simulink model "sampleModel153_pp_1136_1"  (R2021a)
settings: Solver=VariableStepAuto  StartTime=0.0  StopTime=10.0  RelTol=1e-3
undefined symbols (not defined in the file or in its folder): DiscIntNeverNeededParam, magnitude, Newton, Raphson
libraries: simulink x48, pid_lib x19
(part 1 of 3)
settings Model: Creator=CMelt  LastModifiedBy=user

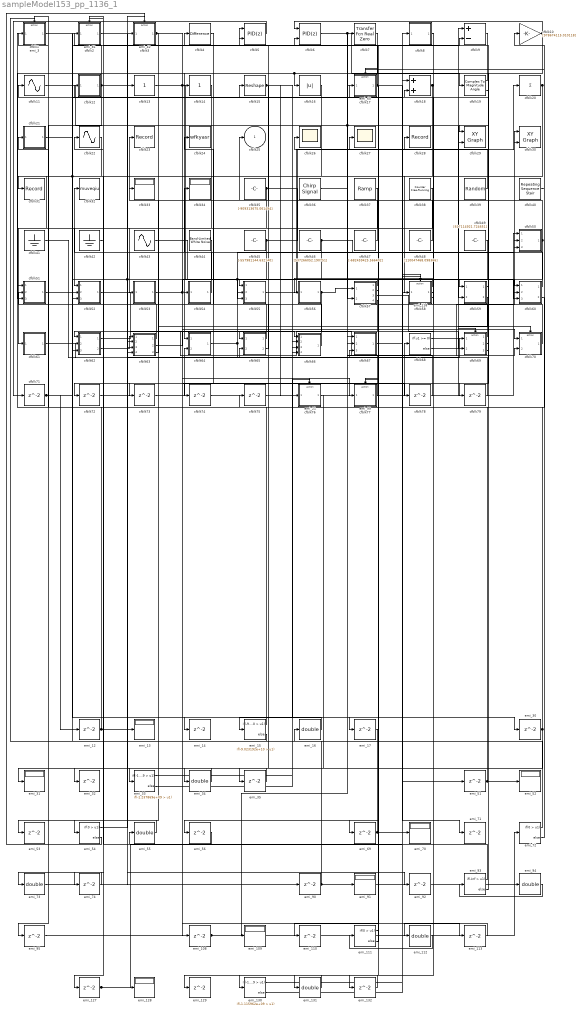
== system sampleModel153_pp_1136_1 ==
  cfblk1 : Subsystem  TreatAsAtomicUnit=on
  cfblk10 : Gain  Gain=[978674115.010118]
  cfblk11 : Sin  TimeSource=Use external signal  SampleTime=0
  cfblk12 : Subsystem  TreatAsAtomicUnit=on
  cfblk13 : simulink/Math Operations/Slider Gain  gain=1  low=0  high=2
  cfblk14 : simulink/Math Operations/Slider Gain  gain=1  low=0  high=2
  cfblk15 : Reshape
  cfblk16 : Abs
  cfblk17 : Subsystem  TreatAsAtomicUnit=on
  cfblk18 : Sum
  cfblk19 : ComplexToMagnitudeAngle
  cfblk2 : Subsystem  TreatAsAtomicUnit=on
  cfblk20 : Sum  Inputs=+
  cfblk21 : Subsystem  TreatAsAtomicUnit=on
  cfblk22 : Sin  TimeSource=Use external signal  SampleTime=0
  cfblk23 : Record  FileSettingsInternal="{\"entries\":[{\"content\":{\"excelSettings\":{\"content\":{},\"type\":\"Streamout.ExcelSettings\"}},\"type\":\"Streamout.FileSettingStorage\",\"uuid\":\"90d3bf4d-074c-419f-bc98-93890882def7\"}],\"packageUris\":[\"http://schema.mathworks.com/mf0/streamout_blocks/R2020a\"],\"version\":\"1.0\"}"  SignalsInternal="{\"entries\":[{\"content\":{\"signals\":[{\"content\":{\"blockPath\":[\"sampleModel153_pp_1136_1/cfblk23\"],\"channel\":[],\"dimensions\":[1],\"domain\":\"samplemodel153_pp_1136_1/cfblk23\",\"lineColor\":\"#64d413\",\"plots\":[1],\"port\":1,\"sid\":[\"\"],\"signalID\":1445323,\"signalName\":\"cfblk47\"},\"type\":\"RecordBlkView.Signal\",\"uuid\":\"54714383-f197-4a3d-9991-f85be281b323\"}]},\"type\":\"RecordBlkView.InputSignals\",\"uuid\":\"544324a9-3e37-4335-a052-9c5c4b19bc85\"}],\"packageUris\":[\"http://schema.mathworks.com/mf0/streamout_blocks/R2020a\"],\"version\":\"1.0\"}"  VisualizationBindings="{\"sparklinesplugin\":{\"info\":[{\"bindingParametersList\":[],\"subplotID\":1}]}}"
  cfblk24 : ToWorkspace  VariableName=wfkyasr  SaveFormat=Timeseries  SampleTime=-1
  cfblk26 : Scope
  cfblk27 : Scope
  cfblk28 : Record  FileSettingsInternal="{\"entries\":[{\"content\":{\"excelSettings\":{\"content\":{},\"type\":\"Streamout.ExcelSettings\"}},\"type\":\"Streamout.FileSettingStorage\",\"uuid\":\"e040c9fa-48bd-4228-9996-6934888816c0\"}],\"packageUris\":[\"http://schema.mathworks.com/mf0/streamout_blocks/R2020a\"],\"version\":\"1.0\"}"  SignalsInternal="{\"entries\":[{\"content\":{\"signals\":[{\"content\":{\"blockPath\":[\"sampleModel153_pp_1136_1/cfblk28\"],\"channel\":[],\"dimensions\":[1],\"domain\":\"samplemodel153_pp_1136_1/cfblk28\",\"lineColor\":\"#a2142f\",\"plots\":[1],\"port\":1,\"sid\":[\"\"],\"signalID\":1445307,\"signalName\":\"cfblk70\"},\"type\":\"RecordBlkView.Signal\",\"uuid\":\"60194e6e-711a-4c83-acfc-41706555a870\"}]},\"type\":\"RecordBlkView.InputSignals\",\"uuid\":\"f9cd218e-cda2-4dab-b38f-344dbdd6f2d9\"}],\"packageUris\":[\"http://schema.mathworks.com/mf0/streamout_blocks/R2020a\"],\"version\":\"1.0\"}"  VisualizationBindings="{\"sparklinesplugin\":{\"info\":[{\"bindingParametersList\":[],\"subplotID\":1}]}}"
  cfblk29 : simulink/Sinks/XY Graph  xmin=-1  xmax=1  ymin=-1  ymax=1  st=-1
  cfblk3 : Subsystem  TreatAsAtomicUnit=on
  cfblk30 : simulink/Sinks/XY Graph  xmin=-1  xmax=1  ymin=-1  ymax=1  st=-1
  cfblk31 : Record  FileSettingsInternal="{\"entries\":[{\"content\":{\"excelSettings\":{\"content\":{},\"type\":\"Streamout.ExcelSettings\"}},\"type\":\"Streamout.FileSettingStorage\",\"uuid\":\"d257a69d-5f58-45b3-980e-d66c6de6435d\"}],\"packageUris\":[\"http://schema.mathworks.com/mf0/streamout_blocks/R2020a\"],\"version\":\"1.0\"}"  SignalsInternal="{\"entries\":[{\"content\":{\"signals\":[{\"content\":{\"blockPath\":[\"sampleModel153_pp_1136_1/cfblk31\"],\"channel\":[],\"dimensions\":[1],\"domain\":\"samplemodel153_pp_1136_1/cfblk31\",\"lineColor\":\"#139fff\",\"plots\":[1],\"port\":1,\"sid\":[\"\"],\"signalID\":1445311,\"signalName\":\"cfblk22\"},\"type\":\"RecordBlkView.Signal\",\"uuid\":\"a9ae145c-d94a-4c8d-ae8c-213f4e7c6313\"}]},\"type\":\"RecordBlkView.InputSignals\",\"uuid\":\"9bb384fc-6cf1-475e-b446-87fd7b0246af\"}],\"packageUris\":[\"http://schema.mathworks.com/mf0/streamout_blocks/R2020a\"],\"version\":\"1.0\"}"  VisualizationBindings="{\"sparklinesplugin\":{\"info\":[{\"bindingParametersList\":[],\"subplotID\":1}]}}"
  cfblk32 : ToWorkspace  VariableName=muveqiu  SaveFormat=Timeseries  SampleTime=-1
  cfblk33 : Display
  cfblk34 : Display
  cfblk35 : Constant  Value=[-909313675.061494]  SampleTime=1
  cfblk36 : simulink/Sources/Chirp Signal  f1=[222988645.109362]  T=[-499288554.133847]  f2=[-768297567.598976]
  cfblk37 : simulink/Sources/Ramp  slope=[-4243.323419]  start=[2.640066]  InitialOutput=[-454218.144588]
  cfblk38 : simulink/Sources/Counter Free-Running  NumBits=[41.000000]  tsamp=-1
  cfblk39 : RandomNumber  Mean=[50925.059613]  Variance=[74743.961687]  Seed=[936037609.000000]  SampleTime=0.1
  cfblk4 : simulink/Discrete/Difference  ICPrevInput=0.0  OutMin=[]  OutMax=[]  OutDataTypeStr=Inherit: Inherit via back propagation  OutDataType=fixdt(1, 16)  OutScaling=2^-10  DoSatur=off
  cfblk40 : simulink/Sources/Repeating Sequence Stair  OutValues=[20471336.287258, 516776994.362484]  tsamp=-1  OutMin=[]  OutMax=[]  OutDataTypeStr=double  OutputDataTypeScalingMode=double  OutDataType=fixdt(0,8)  ConRadixGroup=Best Precision: Vector-wise  OutScaling=2^-12
  cfblk41 : Ground
  cfblk42 : Ground
  cfblk43 : Sin  Amplitude=[411017869.631125]  Bias=[-642889720.785330]  SampleTime=0
  cfblk44 : simulink/Sources/Band-Limited White Noise  Cov=[8221267165.313615]  Ts=0.1  seed=[5325572605.000000]
  cfblk45 : Constant  Value=[-557981144.632140]  SampleTime=1
  cfblk46 : Constant  Value=[537266052.190751]  SampleTime=1
  cfblk47 : Constant  Value=[-682459425.566402]  SampleTime=1
  cfblk48 : Constant  Value=[110047468.098366]  SampleTime=1
  cfblk49 : Constant  Value=[617114921.724651]  SampleTime=1
  cfblk5 : pid_lib/PID Controller (2DOF)  Controller=PID  Form=Parallel  TimeDomain=Discrete-time  UseExternalTs=off  SampleTime=1  IntegratorMethod=Forward Euler  FilterMethod=Forward Euler  ControllerParametersSource=internal  P=1  I=1  D=0  UseFilter=on  N=100  b=1  c=1  TunerSelectOption=Transfer Function Based (PID Tuner App)  InitialConditionSource=internal  InitialConditionForIntegrator=0  InitialConditionForFilter=0  DifferentiatorICPrevScaledInput=0  ExternalReset=none  TrackingMode=off  Kt=1  LimitOutput=off  SatLimitsSource=internal  UpperSaturationLimit=inf  LowerSaturationLimit=-inf  LinearizeAsGain=off  AntiWindupMode=none  Kb=1  POutMin=[]  POutMax=[]  IOutMin=[]  IOutMax=[]  DOutMin=[]  DOutMax=[]  NOutMin=[]  NOutMax=[]  bOutMin=[]  bOutMax=[]  cOutMin=[]  cOutMax=[]  SumOutMin=[]  SumOutMax=[]  SaturationOutMin=[]  SaturationOutMax=[]  PParamMin=[]  PParamMax=[]  IParamMin=[]  IParamMax=[]  DParamMin=[]  DParamMax=[]  NParamMin=[]  NParamMax=[]  bParamMin=[]  bParamMax=[]  cParamMin=[]  cParamMax=[]  KbParamMin=[]  KbParamMax=[]  KtParamMin=[]  KtParamMax=[]  KbOutMin=[]  KbOutMax=[]  KtOutMin=[]  KtOutMax=[]  IntegratorOutMin=[]  IntegratorOutMax=[]  FilterOutMin=[]  FilterOutMax=[]  SumI1OutMin=[]  SumI1OutMax=[]  SumI2OutMin=[]  SumI2OutMax=[]  SumI3OutMin=[]  SumI3OutMax=[]  SumI4OutMin=[]  SumI4OutMax=[]  SumDOutMin=[]  SumDOutMax=[]  Sum1OutMin=[]  Sum1OutMax=[]  Sum2OutMin=[]  Sum2OutMax=[]  Sum3OutMin=[]  Sum3OutMax=[]  DifferentiatorOutMin=[]  DifferentiatorOutMax=[]  FilterDiffOutCoefMin=[]  FilterDiffOutCoefMax=[]  ReciprocalOutMin=[]  ReciprocalOutMax=[]  SumDenOutMin=[]  SumDenOutMax=[]  SumNumOutMin=[]  SumNumOutMax=[]  DivideOutMin=[]  DivideOutMax=[]  UdiffTsProdOutMin=[]  UdiffTsProdOutMax=[]  NTsProdOutMin=[]  NTsProdOutMax=[]  UintegralTsProdOutMin=[]  UintegralTsProdOutMax=[]  UngainTsProdOutMin=[]  UngainTsProdOutMax=[]  IntegratorContinuousStateAttributes=''  IntegratorStateMustResolveToSignalObject=off  IntegratorRTWStateStorageClass=Auto  FilterContinuousStateAttributes=''  FilterStateMustResolveToSignalObject=off  FilterRTWStateStorageClass=Auto  ParallelPVariant=InternalParameters  IdealPVariant=Disabled  IVariant=InternalParameters  DVariant=InternalParameters  bVariant=InternalParameters  cVariant=InternalParameters  IntegratorVariant=Discrete  SatVariant=Disabled  AWVariant=Passthrough  PCopyVariant=Disabled  TRVariant=Disabled  FdbkBlocksVariant=Forward  IdealPFdbkVariant=Disabled  SatFdbkVariant=Disabled  DerivativeFilterVariant=ForwardEulerFilter  NVariant=InternalParameters  NCopyVariant=Disabled  FilterICVariant=InternalICsFilter  IntegratorICVariant=InternalICs  ExternalResetVariant=Disabled  TRSumVariant=Passthrough  SumFdbkVariant=Disabled  SumVariant=Sum_PID  TsampFilterVariant=InternalTs  TsampNgainVariant=Passthrough  TsampIntegralVariant=Passthrough  ExternalSaturationOutDataTypeStr=Inherit: Same as second input
      settings: SourceProductBaseCode=SL
  cfblk50 : Subsystem
  cfblk51 : Subsystem
  cfblk52 : Subsystem
  cfblk53 : Subsystem
  cfblk54 : Subsystem
  cfblk55 : Subsystem
  cfblk56 : Subsystem
  cfblk57 : Subsystem
  cfblk58 : Subsystem  TreatAsAtomicUnit=on
  cfblk59 : Subsystem
  cfblk6 : pid_lib/PID Controller (2DOF)  Controller=PID  Form=Parallel  TimeDomain=Discrete-time  UseExternalTs=off  SampleTime=1  IntegratorMethod=Forward Euler  FilterMethod=Forward Euler  ControllerParametersSource=internal  P=1  I=1  D=0  UseFilter=on  N=100  b=1  c=1  TunerSelectOption=Transfer Function Based (PID Tuner App)  InitialConditionSource=internal  InitialConditionForIntegrator=0  InitialConditionForFilter=0  DifferentiatorICPrevScaledInput=0  ExternalReset=none  TrackingMode=off  Kt=1  LimitOutput=off  SatLimitsSource=internal  UpperSaturationLimit=inf  LowerSaturationLimit=-inf  LinearizeAsGain=off  AntiWindupMode=none  Kb=1  POutMin=[]  POutMax=[]  IOutMin=[]  IOutMax=[]  DOutMin=[]  DOutMax=[]  NOutMin=[]  NOutMax=[]  bOutMin=[]  bOutMax=[]  cOutMin=[]  cOutMax=[]  SumOutMin=[]  SumOutMax=[]  SaturationOutMin=[]  SaturationOutMax=[]  PParamMin=[]  PParamMax=[]  IParamMin=[]  IParamMax=[]  DParamMin=[]  DParamMax=[]  NParamMin=[]  NParamMax=[]  bParamMin=[]  bParamMax=[]  cParamMin=[]  cParamMax=[]  KbParamMin=[]  KbParamMax=[]  KtParamMin=[]  KtParamMax=[]  KbOutMin=[]  KbOutMax=[]  KtOutMin=[]  KtOutMax=[]  IntegratorOutMin=[]  IntegratorOutMax=[]  FilterOutMin=[]  FilterOutMax=[]  SumI1OutMin=[]  SumI1OutMax=[]  SumI2OutMin=[]  SumI2OutMax=[]  SumI3OutMin=[]  SumI3OutMax=[]  SumI4OutMin=[]  SumI4OutMax=[]  SumDOutMin=[]  SumDOutMax=[]  Sum1OutMin=[]  Sum1OutMax=[]  Sum2OutMin=[]  Sum2OutMax=[]  Sum3OutMin=[]  Sum3OutMax=[]  DifferentiatorOutMin=[]  DifferentiatorOutMax=[]  FilterDiffOutCoefMin=[]  FilterDiffOutCoefMax=[]  ReciprocalOutMin=[]  ReciprocalOutMax=[]  SumDenOutMin=[]  SumDenOutMax=[]  SumNumOutMin=[]  SumNumOutMax=[]  DivideOutMin=[]  DivideOutMax=[]  UdiffTsProdOutMin=[]  UdiffTsProdOutMax=[]  NTsProdOutMin=[]  NTsProdOutMax=[]  UintegralTsProdOutMin=[]  UintegralTsProdOutMax=[]  UngainTsProdOutMin=[]  UngainTsProdOutMax=[]  IntegratorContinuousStateAttributes=''  IntegratorStateMustResolveToSignalObject=off  IntegratorRTWStateStorageClass=Auto  FilterContinuousStateAttributes=''  FilterStateMustResolveToSignalObject=off  FilterRTWStateStorageClass=Auto  ParallelPVariant=InternalParameters  IdealPVariant=Disabled  IVariant=InternalParameters  DVariant=InternalParameters  bVariant=InternalParameters  cVariant=InternalParameters  IntegratorVariant=Discrete  SatVariant=Disabled  AWVariant=Passthrough  PCopyVariant=Disabled  TRVariant=Disabled  FdbkBlocksVariant=Forward  IdealPFdbkVariant=Disabled  SatFdbkVariant=Disabled  DerivativeFilterVariant=ForwardEulerFilter  NVariant=InternalParameters  NCopyVariant=Disabled  FilterICVariant=InternalICsFilter  IntegratorICVariant=InternalICs  ExternalResetVariant=Disabled  TRSumVariant=Passthrough  SumFdbkVariant=Disabled  SumVariant=Sum_PID  TsampFilterVariant=InternalTs  TsampNgainVariant=Passthrough  TsampIntegralVariant=Passthrough  ExternalSaturationOutDataTypeStr=Inherit: Same as second input
      settings: SourceProductBaseCode=SL
  cfblk60 : Subsystem
  cfblk61 : Subsystem
  cfblk62 : Subsystem
  cfblk63 : Subsystem
  cfblk64 : Subsystem
  cfblk65 : Subsystem
  cfblk66 : Subsystem
  cfblk67 : Subsystem
  cfblk68 : If  IfExpression=u1 >= 0  SampleTime=1
  cfblk69 : Subsystem  TreatAsAtomicUnit=on
  cfblk7 : simulink/Discrete/Transfer Fcn Real Zero  ZeroZ=0.75  ICPrevInput=0.0  DoSatur=off
      settings: SourceProductBaseCode=SL
  cfblk70 : Subsystem  TreatAsAtomicUnit=on
  cfblk{71..75,78..79} (7 alike) : Delay  SampleTime=1
  cfblk76 : Subsystem  TreatAsAtomicUnit=on
  cfblk77 : Subsystem  TreatAsAtomicUnit=on
  cfblk8 : ModelReference  ModelNameDialog=sampleModel_ref_684  SimulationMode=Normal  ModelReferenceVersion=1.1
  cfblk9 : Sum  Inputs=+-
  emi_{12,14,30,32,90,92,108,110} (8 alike) : Delay
  emi_{13,31,52,70,91,109,128} (7 alike) : Display
  emi_111 : If  IfExpression=0 > u1  SampleTime=1
  emi_{16,34,55,73,94,112,131} (7 alike) : DataTypeConversion  OutDataTypeStr=double
  emi_113 : Delay  InitialCondition=0
  emi_118 : Subsystem  TreatAsAtomicUnit=on
  emi_{51,53,69,71,127,129} (6 alike) : Delay  SampleTime=1
  emi_130 : If  IfExpression=-1.115962e+09 > u1
  emi_132 : Delay  InitialCondition=-557981144.6321
  emi_15 : If  IfExpression=-9.023192e+10 > u1  SampleTime=1
  emi_17 : Delay  InitialCondition=-45115958295.9639
  emi_21 : Subsystem  TreatAsAtomicUnit=on
  emi_3 : Subsystem  TreatAsAtomicUnit=on
  emi_33 : If  IfExpression=-1.237869e+09 > u1  SampleTime=1
  emi_35 : Delay  InitialCondition=-618934691.025
  emi_42 : Subsystem  TreatAsAtomicUnit=on
  emi_54 : If  IfExpression=0 > u1  SampleTime=1
  emi_56 : Delay  InitialCondition=0
  emi_60 : Subsystem  TreatAsAtomicUnit=on
  emi_72 : If  IfExpression=0 > u1
  emi_74 : Delay  InitialCondition=0
  emi_81 : Subsystem  TreatAsAtomicUnit=on
  emi_93 : If  IfExpression=-Inf > u1
  emi_95 : Delay  InitialCondition=-Inf
  emi_99 : Subsystem  TreatAsAtomicUnit=on
  cfblk25 : Outport
  wires:
  cfblk9/1 -> cfblk64/1(cfblk1)
  cfblk47/1 -> cfblk23/1
  cfblk38/1 -> cfblk52/1(cfblk1)
  cfblk57/1(cfblk2) -> cfblk52/2(cfblk8)
  cfblk41/1 -> cfblk69/1(cfblk1)
  cfblk39/1 -> cfblk27/1
  cfblk49/1 -> cfblk54/1(cfblk1)
  cfblk62/1(cfblk2) -> cfblk30/1
  cfblk63/2(cfblk15) -> cfblk66/1(cfblk1)
  cfblk35/1 -> cfblk61/1(cfblk1), cfblk60/2(cfblk10)
  cfblk57/2(cfblk12) -> cfblk11/1
  cfblk22/1 -> cfblk31/1
  cfblk6/1 -> cfblk29/2, cfblk60/3(cfblk11), cfblk19/1
  cfblk48/1 -> cfblk25/1
  cfblk70/1(cfblk2) -> cfblk28/1
  cfblk62/2(cfblk11) -> cfblk63/1(cfblk1)
  cfblk46/1 -> cfblk52/3(cfblk9), cfblk55/3(cfblk12), cfblk50/3(cfblk14)
  cfblk52/1(cfblk2) -> cfblk65/1(cfblk1)
  cfblk13/1 -> cfblk55/1(cfblk1), cfblk70/1(cfblk1)
  cfblk36/1 -> cfblk7/1
  cfblk63/3(cfblk16) -> cfblk33/1
  cfblk54/1(cfblk2) -> cfblk32/1
  cfblk61/1(cfblk2) -> cfblk65/2(cfblk6)
  cfblk19/1 -> cfblk14/1
  cfblk10/1 -> cfblk6/1, cfblk29/1
  cfblk14/1 -> cfblk53/1(cfblk1)
  cfblk66/1(cfblk2) -> cfblk24/1
  cfblk65/1(cfblk2) -> cfblk22/1
  cfblk16/1 -> cfblk51/1(cfblk1), cfblk62/3(cfblk10)
  cfblk37/1 -> cfblk66/2(cfblk12)
  cfblk60/1(cfblk2) -> cfblk34/1
  cfblk7/1 -> cfblk16/1, cfblk51/3(cfblk7)
  cfblk65/2(cfblk7) -> cfblk51/2(cfblk6)
  cfblk57/3(cfblk13) -> cfblk69/2(cfblk10)
  cfblk69/1(cfblk2) -> cfblk4/1
  cfblk53/1(cfblk2) -> cfblk59/1(cfblk1), cfblk78/1
  cfblk11/1 -> cfblk59/2(cfblk6)
  cfblk56/1(cfblk2) -> cfblk57/1(cfblk1), cfblk63/4(cfblk14)
  cfblk55/1(cfblk2) -> cfblk30/2
  cfblk51/1(cfblk2) -> cfblk5/1
  cfblk44/1 -> cfblk63/3(cfblk13), cfblk62/2(cfblk9)
  cfblk69/2(cfblk11) -> cfblk15/1
  cfblk69/3(cfblk12) -> cfblk26/1
  cfblk15/1 -> cfblk60/1(cfblk1), cfblk76/1(emi_19), emi_30/1, emi_35/1
  cfblk40/1 -> cfblk10/1
  cfblk43/1 -> cfblk66/3(cfblk13)
  cfblk64/1(cfblk2) -> cfblk50/2(cfblk13), cfblk67/3(cfblk7)
  cfblk45/1 -> cfblk55/2(cfblk11), cfblk20/1
  cfblk57/4(cfblk14) -> cfblk66/4(cfblk14)
  cfblk50/1(cfblk2) -> cfblk57/2(cfblk11), cfblk5/2
  cfblk68/1 -> cfblk69/Action
  cfblk68/2 -> cfblk70/Action
  cfblk5/1 -> cfblk71/1
  cfblk59/1(cfblk2) -> cfblk72/1
  cfblk72/1 -> cfblk64/2(cfblk7)
  cfblk59/2(cfblk7) -> cfblk73/1
  cfblk73/1 -> cfblk9/1
  cfblk4/1 -> cfblk74/1
  cfblk74/1 -> cfblk68/1
  cfblk60/2(cfblk12) -> cfblk75/1
  cfblk75/1 -> cfblk50/1(cfblk1)
  cfblk78/1 -> cfblk67/2(cfblk6)
  cfblk19/2 -> cfblk79/1
  cfblk79/1 -> cfblk63/2(cfblk12)
  cfblk71/1 -> cfblk1/1(emi_1), emi_12/1, emi_17/1
  cfblk1/1(emi_2) -> cfblk9/2
  emi_12/1 -> emi_3/1(emi_10), emi_13/1
  emi_3/1(emi_11) -> emi_14/1
  emi_15/2 -> cfblk1/Action
  emi_15/1 -> emi_3/Action
  emi_16/1 -> emi_15/1
  emi_17/1 -> emi_16/1
  cfblk76/1(emi_20) -> cfblk70/2(cfblk9)
  emi_30/1 -> emi_21/1(emi_28), emi_31/1
  emi_21/1(emi_29) -> emi_32/1
  emi_33/2 -> cfblk76/Action
  emi_33/1 -> emi_21/Action
  emi_34/1 -> emi_33/1
  emi_35/1 -> emi_34/1
  cfblk42/1 -> cfblk12/1(emi_37)
  cfblk3/1(emi_41) -> cfblk6/2, cfblk77/1(emi_97), emi_108/1, emi_113/1
  emi_51/1 -> emi_42/1(emi_49), emi_52/1
  emi_42/1(emi_50) -> emi_53/1
  emi_54/2 -> cfblk3/Action
  emi_54/1 -> emi_42/Action
  emi_55/1 -> emi_54/1
  emi_56/1 -> emi_55/1
  cfblk18/1 -> cfblk17/1(emi_58), emi_69/1, emi_74/1
  cfblk17/1(emi_59) -> emi_56/1, emi_51/1, cfblk3/1(emi_40)
  emi_69/1 -> emi_60/1(emi_67), emi_70/1
  emi_60/1(emi_68) -> emi_71/1
  emi_72/2 -> cfblk17/Action
  emi_72/1 -> emi_60/Action
  emi_73/1 -> emi_72/1
  emi_74/1 -> emi_73/1
  cfblk63/1(cfblk2) -> cfblk21/1(emi_76)
  cfblk21/1(emi_77) -> cfblk18/1
  cfblk12/1(emi_38) -> cfblk2/1(emi_79), emi_90/1, emi_95/1
  cfblk2/1(emi_80) -> cfblk13/1
  emi_90/1 -> emi_81/1(emi_88), emi_91/1
  emi_81/1(emi_89) -> emi_92/1
  emi_93/2 -> cfblk2/Action
  emi_93/1 -> emi_81/Action
  emi_94/1 -> emi_93/1
  emi_95/1 -> emi_94/1
  cfblk77/1(emi_98) -> cfblk67/1(cfblk1)
  emi_108/1 -> emi_99/1(emi_106), emi_109/1
  emi_99/1(emi_107) -> emi_110/1
  emi_111/2 -> cfblk77/Action
  emi_111/1 -> emi_99/Action
  emi_112/1 -> emi_111/1
  emi_113/1 -> emi_112/1
  cfblk20/1 -> cfblk58/1(emi_115), emi_127/1, emi_132/1
  cfblk58/1(emi_116) -> cfblk56/1(cfblk1)
  cfblk58/2(emi_117) -> cfblk18/2
  emi_127/1 -> emi_118/1(emi_125), emi_128/1
  emi_118/1(emi_126) -> emi_129/1
  emi_130/2 -> cfblk58/Action
  emi_130/1 -> emi_118/Action
  emi_131/1 -> emi_130/1
  emi_132/1 -> emi_131/1
  cfblk67/1(cfblk2) -> cfblk8/1
  cfblk8/1 -> cfblk62/1(cfblk1)

== system sampleModel153_pp_1136_1/cfblk1 ==
  emi_1 : Inport
  Action Port : ActionPort  ActionPortLabel=else
  cfblk1 : DiscreteFir  SampleTime=1
  emi_2 : Outport
  wires:
  emi_1/1 -> cfblk1/1
  cfblk1/1 -> emi_2/1

== system sampleModel153_pp_1136_1/cfblk12 ==
  emi_37 : Inport  Partition=on  PartitionDimension=1  PartitionWidth=1  PartitionOffset=0
  For Each : ForEach  DisableCoverage=on
  cfblk12 : Math  Operator=log10  SaturateOnIntegerOverflow=on
  emi_38 : Outport  ConcatenationDimension=1
  wires:
  emi_37/1 -> cfblk12/1
  cfblk12/1 -> emi_38/1

== system sampleModel153_pp_1136_1/cfblk17 ==
  emi_58 : Inport
  Action Port : ActionPort  ActionPortLabel=else
  cfblk17 : Signum
  emi_59 : Outport
  wires:
  emi_58/1 -> cfblk17/1
  cfblk17/1 -> emi_59/1

== system sampleModel153_pp_1136_1/cfblk2 ==
  emi_79 : Inport
  Action Port : ActionPort  ActionPortLabel=else
  cfblk2 : simulink/Discrete/Difference  ICPrevInput=0.0  OutMin=[]  OutMax=[]  OutDataTypeStr=Inherit: Inherit via back propagation  OutDataType=fixdt(1, 16)  OutScaling=2^-10  DoSatur=off
  emi_80 : Outport
  wires:
  emi_79/1 -> cfblk2/1
  cfblk2/1 -> emi_80/1

== system sampleModel153_pp_1136_1/cfblk21 ==
  emi_76 : Inport  Partition=on  PartitionDimension=1  PartitionWidth=1  PartitionOffset=0
  For Each : ForEach  DisableCoverage=on
  cfblk21 : Rounding
  emi_77 : Outport  ConcatenationDimension=1
  wires:
  emi_76/1 -> cfblk21/1
  cfblk21/1 -> emi_77/1

== system sampleModel153_pp_1136_1/cfblk3 ==
  emi_40 : Inport
  Action Port : ActionPort  ActionPortLabel=else
  cfblk3 : DiscreteFilter  SampleTime=1
  emi_41 : Outport
  wires:
  emi_40/1 -> cfblk3/1
  cfblk3/1 -> emi_41/1

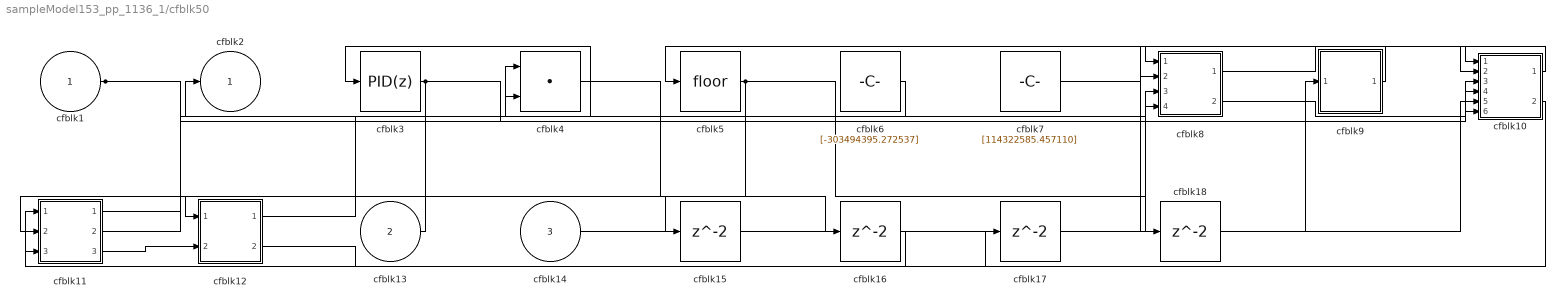
== system sampleModel153_pp_1136_1/cfblk50 ==
  cfblk1 : Inport
  cfblk13 : Inport  Port=2
  cfblk14 : Inport  Port=3
  cfblk10 : Subsystem
  cfblk11 : Subsystem
  cfblk12 : Subsystem
  cfblk{15..18} (4 alike) : Delay  SampleTime=1
  cfblk3 : pid_lib/PID Controller  Controller=PID  Form=Parallel  TimeDomain=Discrete-time  UseExternalTs=off  SampleTime=1  IntegratorMethod=Forward Euler  FilterMethod=Forward Euler  ControllerParametersSource=internal  P=1  I=1  D=0  UseFilter=on  N=100  TunerSelectOption=Transfer Function Based (PID Tuner App)  InitialConditionSource=internal  InitialConditionForIntegrator=0  InitialConditionForFilter=0  DifferentiatorICPrevScaledInput=0  ExternalReset=none  TrackingMode=off  Kt=1  LimitOutput=off  SatLimitsSource=internal  UpperSaturationLimit=inf  LowerSaturationLimit=-inf  LinearizeAsGain=off  AntiWindupMode=none  Kb=1  POutMin=[]  POutMax=[]  IOutMin=[]  IOutMax=[]  DOutMin=[]  DOutMax=[]  NOutMin=[]  NOutMax=[]  SumOutMin=[]  SumOutMax=[]  SaturationOutMin=[]  SaturationOutMax=[]  PParamMin=[]  PParamMax=[]  IParamMin=[]  IParamMax=[]  DParamMin=[]  DParamMax=[]  NParamMin=[]  NParamMax=[]  KbParamMin=[]  KbParamMax=[]  KtParamMin=[]  KtParamMax=[]  KbOutMin=[]  KbOutMax=[]  KtOutMin=[]  KtOutMax=[]  IntegratorOutMin=[]  IntegratorOutMax=[]  FilterOutMin=[]  FilterOutMax=[]  SumI1OutMin=[]  SumI1OutMax=[]  SumI2OutMin=[]  SumI2OutMax=[]  SumI3OutMin=[]  SumI3OutMax=[]  SumI4OutMin=[]  SumI4OutMax=[]  SumDOutMin=[]  SumDOutMax=[]  DifferentiatorOutMin=[]  DifferentiatorOutMax=[]  FilterDiffOutCoefMin=[]  FilterDiffOutCoefMax=[]  ReciprocalOutMin=[]  ReciprocalOutMax=[]  SumDenOutMin=[]  SumDenOutMax=[]  SumNumOutMin=[]  SumNumOutMax=[]  DivideOutMin=[]  DivideOutMax=[]  UdiffTsProdOutMin=[]  UdiffTsProdOutMax=[]  NTsProdOutMin=[]  NTsProdOutMax=[]  UintegralTsProdOutMin=[]  UintegralTsProdOutMax=[]  UngainTsProdOutMin=[]  UngainTsProdOutMax=[]  IntegratorContinuousStateAttributes=''  IntegratorStateMustResolveToSignalObject=off  IntegratorRTWStateStorageClass=Auto  FilterContinuousStateAttributes=''  FilterStateMustResolveToSignalObject=off  FilterRTWStateStorageClass=Auto  ParallelPVariant=InternalParameters  IdealPVariant=Disabled  IVariant=InternalParameters  DVariant=InternalParameters  IntegratorVariant=Discrete  SatVariant=Disabled  AWVariant=Passthrough  PCopyVariant=Disabled  TRVariant=Disabled  FdbkBlocksVariant=Forward  IdealPFdbkVariant=Disabled  SatFdbkVariant=Disabled  DerivativeFilterVariant=ForwardEulerFilter  NVariant=InternalParameters  NCopyVariant=Disabled  FilterICVariant=InternalICsFilter  IntegratorICVariant=InternalICs  ExternalResetVariant=Disabled  TRSumVariant=Passthrough  SumFdbkVariant=Disabled  SumVariant=Sum_PID  TsampFilterVariant=InternalTs  TsampNgainVariant=Passthrough  TsampIntegralVariant=Passthrough  ExternalSaturationOutDataTypeStr=Inherit: Same as second input
  cfblk4 : DotProduct  InputSameDT=on  OutDataTypeStr=Inherit: Inherit via internal rule
  cfblk5 : Rounding
  cfblk6 : Constant  Value=[-303494395.272537]  SampleTime=1
  cfblk7 : Constant  Value=[114322585.457110]  SampleTime=1
  cfblk8 : Subsystem
  cfblk9 : Subsystem
  cfblk2 : Outport
  wires:
  cfblk10/1(cfblk2) -> cfblk5/1
  cfblk14/1 -> cfblk9/1(cfblk1)
  cfblk12/1(cfblk2) -> cfblk4/1
  cfblk10/2(cfblk13) -> cfblk11/1(cfblk1)
  cfblk6/1 -> cfblk3/1
  cfblk3/1 -> cfblk12/1(cfblk1), cfblk10/6(cfblk12)
  cfblk9/1(cfblk2) -> cfblk8/1(cfblk1)
  cfblk5/1 -> cfblk11/2(cfblk12), cfblk18/1
  cfblk13/1 -> cfblk2/1
  cfblk8/1(cfblk2) -> cfblk10/1(cfblk1)
  cfblk7/1 -> cfblk10/2(cfblk8)
  cfblk1/1 -> cfblk8/3(cfblk14), cfblk10/4(cfblk10)
  cfblk8/2(cfblk16) -> cfblk10/3(cfblk9)
  cfblk11/2(cfblk14) -> cfblk4/2
  cfblk11/3(cfblk15) -> cfblk12/2(cfblk6)
  cfblk11/1(cfblk2) -> cfblk15/1
  cfblk15/1 -> cfblk8/4(cfblk15)
  cfblk4/1 -> cfblk16/1
  cfblk16/1 -> cfblk11/3(cfblk13)
  cfblk12/2(cfblk7) -> cfblk17/1
  cfblk17/1 -> cfblk8/2(cfblk13)
  cfblk18/1 -> cfblk10/5(cfblk11)

== system sampleModel153_pp_1136_1/cfblk51 ==
  cfblk1 : Inport
  cfblk6 : Inport  Port=2
  cfblk7 : Inport  Port=3
  cfblk3 : Delay  DelayLengthSource=Input port  SampleTime=1
      settings: InputPortMap=u0,p1
  cfblk4 : Gain  Gain=[295349995.525931]
  cfblk5 : Constant  Value=[-765488157.725793]  SampleTime=1
  cfblk2 : Outport
  wires:
  cfblk1/1 -> cfblk4/1
  cfblk5/1 -> cfblk2/1
  cfblk4/1 -> cfblk3/1
  cfblk7/1 -> cfblk3/2

== system sampleModel153_pp_1136_1/cfblk52 ==
  cfblk1 : Inport
  cfblk8 : Inport  Port=2
  cfblk9 : Inport  Port=3
  cfblk10 : Delay  SampleTime=1
  cfblk11 : Delay  SampleTime=1
  cfblk3 : simulink/Discrete/Transfer Fcn Real Zero  ZeroZ=0.75  ICPrevInput=0.0  DoSatur=off
      settings: SourceProductBaseCode=SL
  cfblk4 : Product  Inputs=**
  cfblk5 : DotProduct  InputSameDT=on  OutDataTypeStr=Inherit: Inherit via internal rule
  cfblk6 : Gain  Gain=[545946883.436725]
  cfblk7 : Subsystem
  cfblk2 : Outport
  wires:
  cfblk6/1 -> cfblk7/2(cfblk12)
  cfblk1/1 -> cfblk6/1, cfblk7/4(cfblk14)
  cfblk3/1 -> cfblk5/1, cfblk11/1
  cfblk9/1 -> cfblk7/3(cfblk13)
  cfblk8/1 -> cfblk5/2
  cfblk4/1 -> cfblk3/1
  cfblk7/1(cfblk2) -> cfblk2/1
  cfblk7/2(cfblk16) -> cfblk4/1, cfblk4/2
  cfblk5/1 -> cfblk10/1
  cfblk10/1 -> cfblk7/1(cfblk1)
  cfblk11/1 -> cfblk7/5(cfblk15)

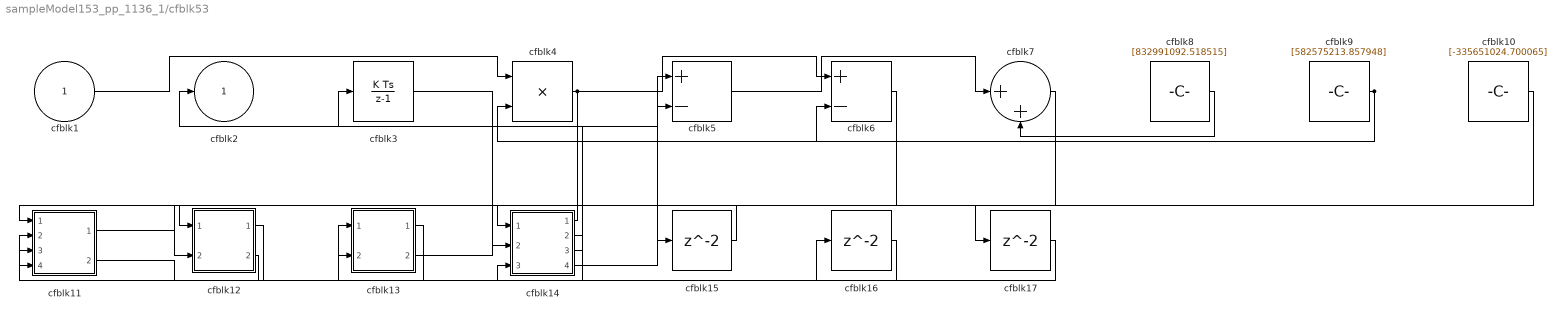
== system sampleModel153_pp_1136_1/cfblk53 ==
  cfblk1 : Inport
  cfblk10 : Constant  Value=[-335651024.700065]  SampleTime=1
  cfblk11 : Subsystem
  cfblk12 : Subsystem
  cfblk13 : Subsystem
  cfblk14 : Subsystem
  cfblk15 : Delay  SampleTime=1
  cfblk16 : Delay  SampleTime=1
  cfblk17 : Delay  SampleTime=1
  cfblk3 : DiscreteIntegrator  ICPrevOutput=DiscIntNeverNeededParam  ICPrevScaledInput=DiscIntNeverNeededParam
  cfblk4 : Product
  cfblk5 : Sum  Inputs=+-
  cfblk6 : Sum  Inputs=+-
  cfblk7 : Sum  Inputs=|++
  cfblk8 : Constant  Value=[832991092.518515]  SampleTime=1
  cfblk9 : Constant  Value=[582575213.857948]  SampleTime=1
  cfblk2 : Outport
  wires:
  cfblk7/1 -> cfblk11/1(cfblk1)
  cfblk14/1(cfblk2) -> cfblk2/1
  cfblk5/1 -> cfblk7/1
  cfblk8/1 -> cfblk7/2
  cfblk4/1 -> cfblk6/1, cfblk12/2(cfblk16)
  cfblk12/1(cfblk2) -> cfblk11/2(cfblk9)
  cfblk6/1 -> cfblk14/1(cfblk1)
  cfblk12/2(cfblk17) -> cfblk11/3(cfblk10)
  cfblk1/1 -> cfblk4/1
  cfblk14/2(cfblk8) -> cfblk13/1(cfblk1)
  cfblk13/1(cfblk2) -> cfblk11/4(cfblk11)
  cfblk10/1 -> cfblk12/1(cfblk1)
  cfblk9/1 -> cfblk6/2, cfblk4/2
  cfblk14/3(cfblk9) -> cfblk3/1
  cfblk14/4(cfblk10) -> cfblk5/1
  cfblk13/2(cfblk13) -> cfblk5/2
  cfblk11/1(cfblk2) -> cfblk15/1
  cfblk15/1 -> cfblk14/2(cfblk6)
  cfblk11/2(cfblk12) -> cfblk16/1
  cfblk16/1 -> cfblk13/2(cfblk12)
  cfblk3/1 -> cfblk17/1
  cfblk17/1 -> cfblk14/3(cfblk7)

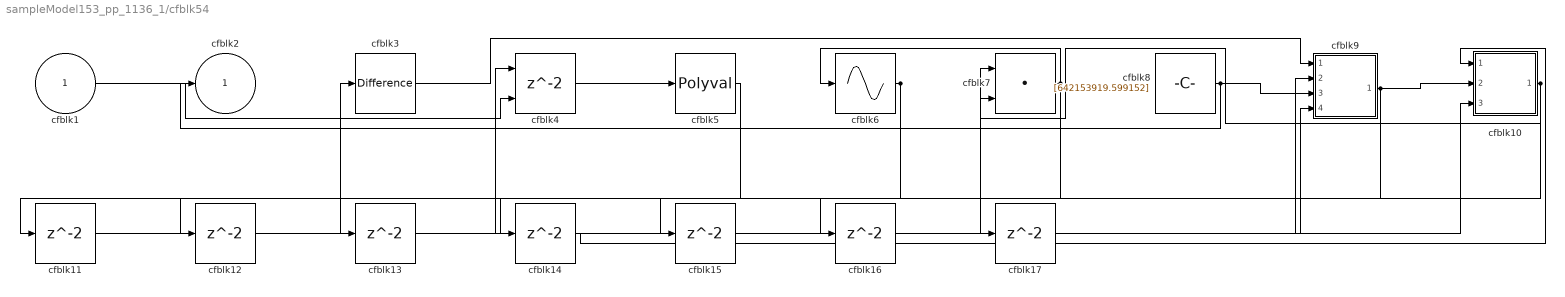
== system sampleModel153_pp_1136_1/cfblk54 ==
  cfblk1 : Inport
  cfblk10 : Subsystem
  cfblk{11..17} (7 alike) : Delay  SampleTime=1
  cfblk3 : simulink/Discrete/Difference  ICPrevInput=0.0  OutMin=[]  OutMax=[]  OutDataTypeStr=Inherit: Inherit via back propagation  OutDataType=fixdt(1, 16)  OutScaling=2^-10  DoSatur=off
  cfblk4 : Delay  ShowEnablePort=on  SampleTime=1
      settings: InputPortMap=u0,e6
  cfblk5 : Polyval  Coefs=[ +2.081618890e-019, -1.441693666e-014, +4.719686976e-010, -8.536869453e-006, +1.621573104e-001, -8.087801117e+001 ]
  cfblk6 : Sin  TimeSource=Use external signal  SampleTime=0
  cfblk7 : DotProduct  InputSameDT=on  OutDataTypeStr=Inherit: Inherit via internal rule
  cfblk8 : Constant  Value=[642153919.599152]  SampleTime=1
  cfblk9 : Subsystem
  cfblk2 : Outport
  wires:
  cfblk1/1 -> cfblk4/2
  cfblk7/1 -> cfblk6/1, cfblk16/1
  cfblk3/1 -> cfblk9/1(cfblk1)
  cfblk8/1 -> cfblk2/1, cfblk9/3(cfblk8)
  cfblk10/1(cfblk2) -> cfblk7/1, cfblk17/1
  cfblk4/1 -> cfblk5/1
  cfblk6/1 -> cfblk13/1, cfblk14/1, cfblk15/1
  cfblk9/1(cfblk2) -> cfblk10/2(cfblk6), cfblk12/1
  cfblk5/1 -> cfblk11/1
  cfblk11/1 -> cfblk4/1
  cfblk12/1 -> cfblk3/1
  cfblk13/1 -> cfblk7/2
  cfblk14/1 -> cfblk10/1(cfblk1)
  cfblk15/1 -> cfblk9/2(cfblk7)
  cfblk16/1 -> cfblk10/3(cfblk7)
  cfblk17/1 -> cfblk9/4(cfblk9)

== system sampleModel153_pp_1136_1/cfblk55 ==
  cfblk1 : Inport
  cfblk11 : Inport  Port=2
  cfblk12 : Inport  Port=3
  cfblk10 : Subsystem
  cfblk13 : Delay  SampleTime=1
  cfblk14 : Delay  SampleTime=1
  cfblk3 : simulink/Discrete/Tapped Delay  vinit=0.0  samptime=-1  NumDelays=1  DelayOrder=Oldest  includeCurrent=off
  cfblk4 : Sum  Inputs=|++
  cfblk5 : ComplexToMagnitudeAngle
  cfblk6 : Assignment  DiagnosticForDimensions=Warning  IndexOptions=Index vector (dialog)  Indices=1  OutputSizes=1
  cfblk7 : Subsystem
  cfblk8 : Subsystem
  cfblk9 : Subsystem
  cfblk2 : Outport
  wires:
  cfblk12/1 -> cfblk4/1
  cfblk6/1 -> cfblk2/1
  cfblk4/1 -> cfblk9/6(cfblk13), cfblk14/1
  cfblk10/1(cfblk2) -> cfblk3/1, cfblk8/2(cfblk9)
  cfblk9/1(cfblk2) -> cfblk6/1
  cfblk11/1 -> cfblk7/1(cfblk1), cfblk9/4(cfblk11)
  cfblk7/1(cfblk2) -> cfblk9/1(cfblk1)
  cfblk1/1 -> cfblk10/2(cfblk8)
  cfblk7/2(cfblk13) -> cfblk9/2(cfblk9), cfblk9/5(cfblk12)
  cfblk3/1 -> cfblk5/1, cfblk7/4(cfblk11)
  cfblk5/1 -> cfblk8/1(cfblk1)
  cfblk5/2 -> cfblk9/3(cfblk10)
  cfblk8/1(cfblk2) -> cfblk7/3(cfblk10)
  cfblk8/2(cfblk10) -> cfblk4/2
  cfblk8/3(cfblk11) -> cfblk6/2, cfblk7/5(cfblk12)
  cfblk9/2(cfblk14) -> cfblk13/1
  cfblk13/1 -> cfblk7/2(cfblk9)
  cfblk14/1 -> cfblk10/1(cfblk1)

== system sampleModel153_pp_1136_1/cfblk56 ==
  cfblk1 : Inport
  cfblk3 : UnitDelay  HasFrameUpgradeWarning=on
  cfblk4 : Sum
  cfblk5 : Sqrt  SaturateOnIntegerOverflow=on
  cfblk6 : Constant  Value=[107790846.039973]  SampleTime=1
  cfblk7 : Subsystem
  cfblk8 : Delay  SampleTime=1
  cfblk2 : Outport
  wires:
  cfblk1/1 -> cfblk4/1, cfblk7/3(cfblk11)
  cfblk4/1 -> cfblk5/1, cfblk3/1
  cfblk7/1(cfblk2) -> cfblk2/1
  cfblk6/1 -> cfblk7/1(cfblk1)
  cfblk5/1 -> cfblk7/2(cfblk10), cfblk7/4(cfblk12), cfblk7/5(cfblk13)
  cfblk3/1 -> cfblk8/1
  cfblk8/1 -> cfblk4/2

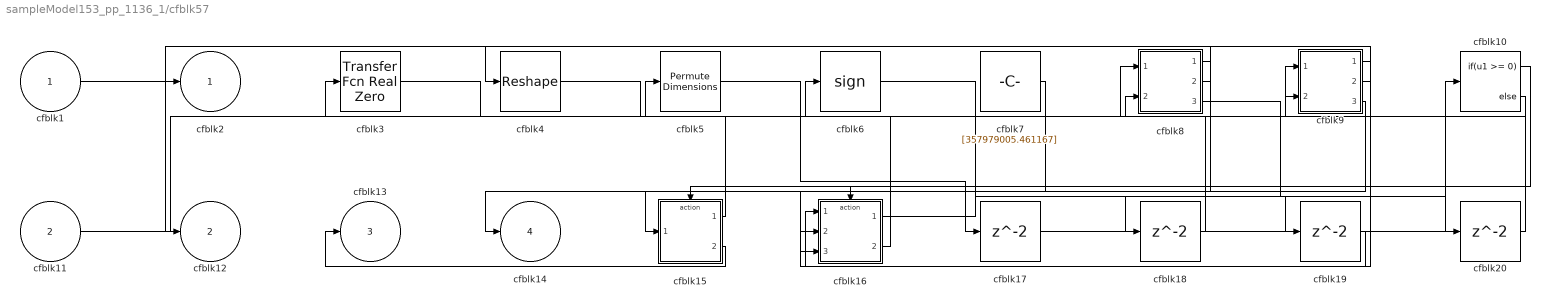
== system sampleModel153_pp_1136_1/cfblk57 ==
  cfblk1 : Inport
  cfblk11 : Inport  Port=2
  cfblk10 : If  IfExpression=u1 >= 0  SampleTime=1
  cfblk15 : Subsystem  TreatAsAtomicUnit=on
  cfblk16 : Subsystem  TreatAsAtomicUnit=on
  cfblk{17..20} (4 alike) : Delay  SampleTime=1
  cfblk3 : simulink/Discrete/Transfer Fcn Real Zero  ZeroZ=0.75  ICPrevInput=0.0  DoSatur=off
      settings: SourceProductBaseCode=SL
  cfblk4 : Reshape
  cfblk5 : PermuteDimensions
  cfblk6 : Signum
  cfblk7 : Constant  Value=[357979005.461167]  SampleTime=1
  cfblk8 : Subsystem
  cfblk9 : Subsystem
  cfblk2 : Outport
  cfblk12 : Outport  Port=2
  cfblk13 : Outport  Port=3
  cfblk14 : Outport  Port=4
  wires:
  cfblk11/1 -> cfblk9/1(cfblk1)
  cfblk1/1 -> cfblk12/1
  cfblk8/1(cfblk2) -> cfblk15/1(cfblk1)
  cfblk15/1(cfblk2) -> cfblk5/1
  cfblk16/2(cfblk12) -> cfblk6/1
  cfblk4/1 -> cfblk9/2(cfblk9)
  cfblk7/1 -> cfblk14/1
  cfblk15/2(cfblk15) -> cfblk13/1
  cfblk8/2(cfblk12) -> cfblk4/1
  cfblk9/1(cfblk2) -> cfblk16/1(cfblk1)
  cfblk3/1 -> cfblk8/2(cfblk11)
  cfblk9/2(cfblk10) -> cfblk2/1
  cfblk9/3(cfblk11) -> cfblk16/3(cfblk11)
  cfblk10/1 -> cfblk15/Action
  cfblk10/2 -> cfblk16/Action
  cfblk5/1 -> cfblk17/1
  cfblk17/1 -> cfblk10/1
  cfblk16/1(cfblk2) -> cfblk18/1
  cfblk18/1 -> cfblk8/1(cfblk1)
  cfblk6/1 -> cfblk19/1
  cfblk19/1 -> cfblk16/2(cfblk10)
  cfblk8/3(cfblk13) -> cfblk20/1
  cfblk20/1 -> cfblk3/1

== system sampleModel153_pp_1136_1/cfblk58 ==
  emi_115 : Inport
  Action Port : ActionPort  ActionPortLabel=else
  cfblk58 : Subsystem
  emi_116 : Outport
  emi_117 : Outport  Port=2
  wires:
  emi_115/1 -> cfblk58/1(cfblk1)
  cfblk58/1(cfblk2) -> emi_116/1
  cfblk58/2(cfblk10) -> emi_117/1

== system sampleModel153_pp_1136_1/cfblk59 ==
  cfblk1 : Inport
  cfblk6 : Inport  Port=2
  cfblk3 : simulink/Math Operations/MinMax Running Resettable  Function=min  vinit=0.0
  cfblk4 : Constant  Value=[-6326451.901417]  SampleTime=1
  cfblk5 : Constant  Value=[640516679.583532]  SampleTime=1
  cfblk2 : Outport
  cfblk7 : Outport  Port=2
  wires:
  cfblk1/1 -> cfblk3/1
  cfblk4/1 -> cfblk2/1
  cfblk3/1 -> cfblk7/1
  cfblk6/1 -> cfblk3/2

== system sampleModel153_pp_1136_1/cfblk60 ==
  cfblk1 : Inport
  cfblk10 : Inport  Port=2
  cfblk11 : Inport  Port=3
  cfblk13 : Delay  SampleTime=1
  cfblk14 : Delay  SampleTime=1
  cfblk3 : pid_lib/PID Controller (2DOF)  Controller=PID  Form=Parallel  TimeDomain=Discrete-time  UseExternalTs=off  SampleTime=1  IntegratorMethod=Forward Euler  FilterMethod=Forward Euler  ControllerParametersSource=internal  P=1  I=1  D=0  UseFilter=on  N=100  b=1  c=1  TunerSelectOption=Transfer Function Based (PID Tuner App)  InitialConditionSource=internal  InitialConditionForIntegrator=0  InitialConditionForFilter=0  DifferentiatorICPrevScaledInput=0  ExternalReset=none  TrackingMode=off  Kt=1  LimitOutput=off  SatLimitsSource=internal  UpperSaturationLimit=inf  LowerSaturationLimit=-inf  LinearizeAsGain=off  AntiWindupMode=none  Kb=1  POutMin=[]  POutMax=[]  IOutMin=[]  IOutMax=[]  DOutMin=[]  DOutMax=[]  NOutMin=[]  NOutMax=[]  bOutMin=[]  bOutMax=[]  cOutMin=[]  cOutMax=[]  SumOutMin=[]  SumOutMax=[]  SaturationOutMin=[]  SaturationOutMax=[]  PParamMin=[]  PParamMax=[]  IParamMin=[]  IParamMax=[]  DParamMin=[]  DParamMax=[]  NParamMin=[]  NParamMax=[]  bParamMin=[]  bParamMax=[]  cParamMin=[]  cParamMax=[]  KbParamMin=[]  KbParamMax=[]  KtParamMin=[]  KtParamMax=[]  KbOutMin=[]  KbOutMax=[]  KtOutMin=[]  KtOutMax=[]  IntegratorOutMin=[]  IntegratorOutMax=[]  FilterOutMin=[]  FilterOutMax=[]  SumI1OutMin=[]  SumI1OutMax=[]  SumI2OutMin=[]  SumI2OutMax=[]  SumI3OutMin=[]  SumI3OutMax=[]  SumI4OutMin=[]  SumI4OutMax=[]  SumDOutMin=[]  SumDOutMax=[]  Sum1OutMin=[]  Sum1OutMax=[]  Sum2OutMin=[]  Sum2OutMax=[]  Sum3OutMin=[]  Sum3OutMax=[]  DifferentiatorOutMin=[]  DifferentiatorOutMax=[]  FilterDiffOutCoefMin=[]  FilterDiffOutCoefMax=[]  ReciprocalOutMin=[]  ReciprocalOutMax=[]  SumDenOutMin=[]  SumDenOutMax=[]  SumNumOutMin=[]  SumNumOutMax=[]  DivideOutMin=[]  DivideOutMax=[]  UdiffTsProdOutMin=[]  UdiffTsProdOutMax=[]  NTsProdOutMin=[]  NTsProdOutMax=[]  UintegralTsProdOutMin=[]  UintegralTsProdOutMax=[]  UngainTsProdOutMin=[]  UngainTsProdOutMax=[]  IntegratorContinuousStateAttributes=''  IntegratorStateMustResolveToSignalObject=off  IntegratorRTWStateStorageClass=Auto  FilterContinuousStateAttributes=''  FilterStateMustResolveToSignalObject=off  FilterRTWStateStorageClass=Auto  ParallelPVariant=InternalParameters  IdealPVariant=Disabled  IVariant=InternalParameters  DVariant=InternalParameters  bVariant=InternalParameters  cVariant=InternalParameters  IntegratorVariant=Discrete  SatVariant=Disabled  AWVariant=Passthrough  PCopyVariant=Disabled  TRVariant=Disabled  FdbkBlocksVariant=Forward  IdealPFdbkVariant=Disabled  SatFdbkVariant=Disabled  DerivativeFilterVariant=ForwardEulerFilter  NVariant=InternalParameters  NCopyVariant=Disabled  FilterICVariant=InternalICsFilter  IntegratorICVariant=InternalICs  ExternalResetVariant=Disabled  TRSumVariant=Passthrough  SumFdbkVariant=Disabled  SumVariant=Sum_PID  TsampFilterVariant=InternalTs  TsampNgainVariant=Passthrough  TsampIntegralVariant=Passthrough  ExternalSaturationOutDataTypeStr=Inherit: Same as second input
      settings: SourceProductBaseCode=SL
  cfblk4 : DiscreteTransferFcn  SampleTime=1
  cfblk5 : DiscreteStateSpace
  cfblk6 : Constant  Value=[-46395399.343327]  SampleTime=1
  cfblk7 : Constant  Value=[-189279799.352586]  SampleTime=1
  cfblk8 : Subsystem
  cfblk9 : Subsystem
  cfblk2 : Outport
  cfblk12 : Outport  Port=2
  wires:
  cfblk8/1(cfblk2) -> cfblk5/1
  cfblk5/1 -> cfblk9/1(cfblk1)
  cfblk4/1 -> cfblk8/1(cfblk1)
  cfblk3/1 -> cfblk4/1
  cfblk7/1 -> cfblk3/2
  cfblk1/1 -> cfblk12/1
  cfblk6/1 -> cfblk8/2(cfblk6)
  cfblk10/1 -> cfblk9/2(cfblk10)
  cfblk11/1 -> cfblk9/3(cfblk11)
  cfblk9/3(cfblk13) -> cfblk2/1
  cfblk9/1(cfblk2) -> cfblk13/1
  cfblk13/1 -> cfblk3/1
  cfblk9/2(cfblk12) -> cfblk14/1
  cfblk14/1 -> cfblk8/3(cfblk7)

== system sampleModel153_pp_1136_1/cfblk61 ==
  cfblk1 : Inport
  cfblk10 : Delay  SampleTime=1
  cfblk11 : Delay  SampleTime=1
  cfblk12 : Delay  SampleTime=1
  cfblk3 : DiscreteZeroPole  Poles=[0 0.5]  Gain=1
  cfblk4 : DiscreteTransferFcn  SampleTime=1
  cfblk5 : Sum  Inputs=+
  cfblk6 : Squeeze
  cfblk7 : Bias  Bias=[62400367.037937]
  cfblk8 : Assignment  DiagnosticForDimensions=Warning  IndexOptions=Index vector (dialog)  Indices=1  OutputSizes=1
  cfblk9 : Subsystem
  cfblk2 : Outport
  wires:
  cfblk5/1 -> cfblk6/1
  cfblk9/1(cfblk2) -> cfblk5/1
  cfblk8/1 -> cfblk9/1(cfblk1)
  cfblk6/1 -> cfblk3/1, cfblk11/1
  cfblk1/1 -> cfblk2/1, cfblk8/2, cfblk9/3(cfblk11)
  cfblk4/1 -> cfblk7/1, cfblk9/2(cfblk10)
  cfblk3/1 -> cfblk10/1
  cfblk10/1 -> cfblk8/1
  cfblk11/1 -> cfblk9/4(cfblk12)
  cfblk7/1 -> cfblk12/1
  cfblk12/1 -> cfblk4/1

== system sampleModel153_pp_1136_1/cfblk62 ==
  cfblk1 : Inport
  cfblk9 : Inport  Port=2
  cfblk10 : Inport  Port=3
  cfblk3 : pid_lib/PID Controller (2DOF)  Controller=PID  Form=Parallel  TimeDomain=Discrete-time  UseExternalTs=off  SampleTime=1  IntegratorMethod=Forward Euler  FilterMethod=Forward Euler  ControllerParametersSource=internal  P=1  I=1  D=0  UseFilter=on  N=100  b=1  c=1  TunerSelectOption=Transfer Function Based (PID Tuner App)  InitialConditionSource=internal  InitialConditionForIntegrator=0  InitialConditionForFilter=0  DifferentiatorICPrevScaledInput=0  ExternalReset=none  TrackingMode=off  Kt=1  LimitOutput=off  SatLimitsSource=internal  UpperSaturationLimit=inf  LowerSaturationLimit=-inf  LinearizeAsGain=off  AntiWindupMode=none  Kb=1  POutMin=[]  POutMax=[]  IOutMin=[]  IOutMax=[]  DOutMin=[]  DOutMax=[]  NOutMin=[]  NOutMax=[]  bOutMin=[]  bOutMax=[]  cOutMin=[]  cOutMax=[]  SumOutMin=[]  SumOutMax=[]  SaturationOutMin=[]  SaturationOutMax=[]  PParamMin=[]  PParamMax=[]  IParamMin=[]  IParamMax=[]  DParamMin=[]  DParamMax=[]  NParamMin=[]  NParamMax=[]  bParamMin=[]  bParamMax=[]  cParamMin=[]  cParamMax=[]  KbParamMin=[]  KbParamMax=[]  KtParamMin=[]  KtParamMax=[]  KbOutMin=[]  KbOutMax=[]  KtOutMin=[]  KtOutMax=[]  IntegratorOutMin=[]  IntegratorOutMax=[]  FilterOutMin=[]  FilterOutMax=[]  SumI1OutMin=[]  SumI1OutMax=[]  SumI2OutMin=[]  SumI2OutMax=[]  SumI3OutMin=[]  SumI3OutMax=[]  SumI4OutMin=[]  SumI4OutMax=[]  SumDOutMin=[]  SumDOutMax=[]  Sum1OutMin=[]  Sum1OutMax=[]  Sum2OutMin=[]  Sum2OutMax=[]  Sum3OutMin=[]  Sum3OutMax=[]  DifferentiatorOutMin=[]  DifferentiatorOutMax=[]  FilterDiffOutCoefMin=[]  FilterDiffOutCoefMax=[]  ReciprocalOutMin=[]  ReciprocalOutMax=[]  SumDenOutMin=[]  SumDenOutMax=[]  SumNumOutMin=[]  SumNumOutMax=[]  DivideOutMin=[]  DivideOutMax=[]  UdiffTsProdOutMin=[]  UdiffTsProdOutMax=[]  NTsProdOutMin=[]  NTsProdOutMax=[]  UintegralTsProdOutMin=[]  UintegralTsProdOutMax=[]  UngainTsProdOutMin=[]  UngainTsProdOutMax=[]  IntegratorContinuousStateAttributes=''  IntegratorStateMustResolveToSignalObject=off  IntegratorRTWStateStorageClass=Auto  FilterContinuousStateAttributes=''  FilterStateMustResolveToSignalObject=off  FilterRTWStateStorageClass=Auto  ParallelPVariant=InternalParameters  IdealPVariant=Disabled  IVariant=InternalParameters  DVariant=InternalParameters  bVariant=InternalParameters  cVariant=InternalParameters  IntegratorVariant=Discrete  SatVariant=Disabled  AWVariant=Passthrough  PCopyVariant=Disabled  TRVariant=Disabled  FdbkBlocksVariant=Forward  IdealPFdbkVariant=Disabled  SatFdbkVariant=Disabled  DerivativeFilterVariant=ForwardEulerFilter  NVariant=InternalParameters  NCopyVariant=Disabled  FilterICVariant=InternalICsFilter  IntegratorICVariant=InternalICs  ExternalResetVariant=Disabled  TRSumVariant=Passthrough  SumFdbkVariant=Disabled  SumVariant=Sum_PID  TsampFilterVariant=InternalTs  TsampNgainVariant=Passthrough  TsampIntegralVariant=Passthrough  ExternalSaturationOutDataTypeStr=Inherit: Same as second input
      settings: SourceProductBaseCode=SL
  cfblk4 : DiscreteZeroPole  Poles=[0 0.5]  Gain=1
  cfblk5 : Squeeze
  cfblk6 : Signum
  cfblk7 : Constant  Value=[877030335.208423]  SampleTime=1
  cfblk8 : Constant  Value=[462418889.977943]  SampleTime=1
  cfblk2 : Outport
  cfblk11 : Outport  Port=2
  wires:
  cfblk10/1 -> cfblk5/1
  cfblk4/1 -> cfblk11/1
  cfblk5/1 -> cfblk2/1
  cfblk9/1 -> cfblk6/1
  cfblk1/1 -> cfblk3/1
  cfblk6/1 -> cfblk4/1
  cfblk7/1 -> cfblk3/2

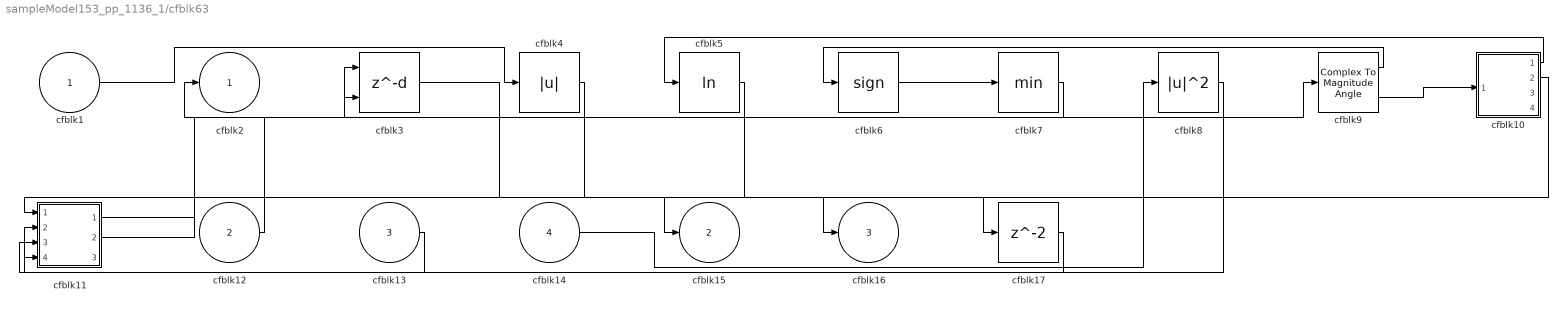
== system sampleModel153_pp_1136_1/cfblk63 ==
  cfblk1 : Inport
  cfblk12 : Inport  Port=2
  cfblk13 : Inport  Port=3
  cfblk14 : Inport  Port=4
  cfblk10 : Subsystem
  cfblk11 : Subsystem
  cfblk17 : Delay  SampleTime=1
  cfblk3 : Delay  DelayLengthSource=Input port  SampleTime=1
      settings: InputPortMap=u0,p1
  cfblk4 : Abs
  cfblk5 : Math  Operator=log  SaturateOnIntegerOverflow=on
  cfblk6 : Signum
  cfblk7 : MinMax
  cfblk8 : Math  Operator=magnitude^2  SaturateOnIntegerOverflow=on
  cfblk9 : ComplexToMagnitudeAngle
  cfblk2 : Outport
  cfblk15 : Outport  Port=2
  cfblk16 : Outport  Port=3
  wires:
  cfblk4/1 -> cfblk11/1(cfblk1)
  cfblk12/1 -> cfblk2/1
  cfblk1/1 -> cfblk4/1
  cfblk8/1 -> cfblk11/2(cfblk10)
  cfblk9/1 -> cfblk6/1
  cfblk5/1 -> cfblk15/1
  cfblk10/1(cfblk2) -> cfblk5/1
  cfblk14/1 -> cfblk8/1
  cfblk9/2 -> cfblk10/1(cfblk1)
  cfblk11/1(cfblk2) -> cfblk9/1
  cfblk11/2(cfblk13) -> cfblk3/1
  cfblk6/1 -> cfblk7/1
  cfblk10/2(cfblk13) -> cfblk16/1
  cfblk7/1 -> cfblk3/2
  cfblk13/1 -> cfblk11/4(cfblk12)
  cfblk3/1 -> cfblk17/1
  cfblk17/1 -> cfblk11/3(cfblk11)

== system sampleModel153_pp_1136_1/cfblk64 ==
  cfblk1 : Inport
  cfblk7 : Inport  Port=2
  cfblk10 : Delay  SampleTime=1
  cfblk3 : Sum  Inputs=+-
  cfblk4 : Product  Inputs=**
  cfblk5 : Product  Inputs=*
  cfblk6 : Subsystem
  cfblk8 : Delay  SampleTime=1
  cfblk9 : Delay  SampleTime=1
  cfblk2 : Outport
  wires:
  cfblk3/1 -> cfblk5/1
  cfblk6/1(cfblk2) -> cfblk4/1
  cfblk7/1 -> cfblk6/1(cfblk1)
  cfblk6/2(cfblk10) -> cfblk4/2
  cfblk1/1 -> cfblk2/1
  cfblk5/1 -> cfblk6/3(cfblk9), cfblk8/1
  cfblk8/1 -> cfblk3/1
  cfblk4/1 -> cfblk9/1
  cfblk9/1 -> cfblk6/2(cfblk8)
  cfblk6/3(cfblk11) -> cfblk10/1
  cfblk10/1 -> cfblk3/2

== system sampleModel153_pp_1136_1/cfblk65 ==
  cfblk1 : Inport
  cfblk6 : Inport  Port=2
  cfblk3 : DiscreteStateSpace
  cfblk4 : Bias  Bias=[709750677.101667]
  cfblk5 : Subsystem
  cfblk8 : Delay  SampleTime=1
  cfblk2 : Outport
  cfblk7 : Outport  Port=2
  wires:
  cfblk5/1(cfblk2) -> cfblk4/1
  cfblk3/1 -> cfblk2/1, cfblk5/3(cfblk10), cfblk5/4(cfblk11)
  cfblk6/1 -> cfblk7/1, cfblk5/2(cfblk9)
  cfblk1/1 -> cfblk3/1
  cfblk4/1 -> cfblk8/1
  cfblk8/1 -> cfblk5/1(cfblk1)

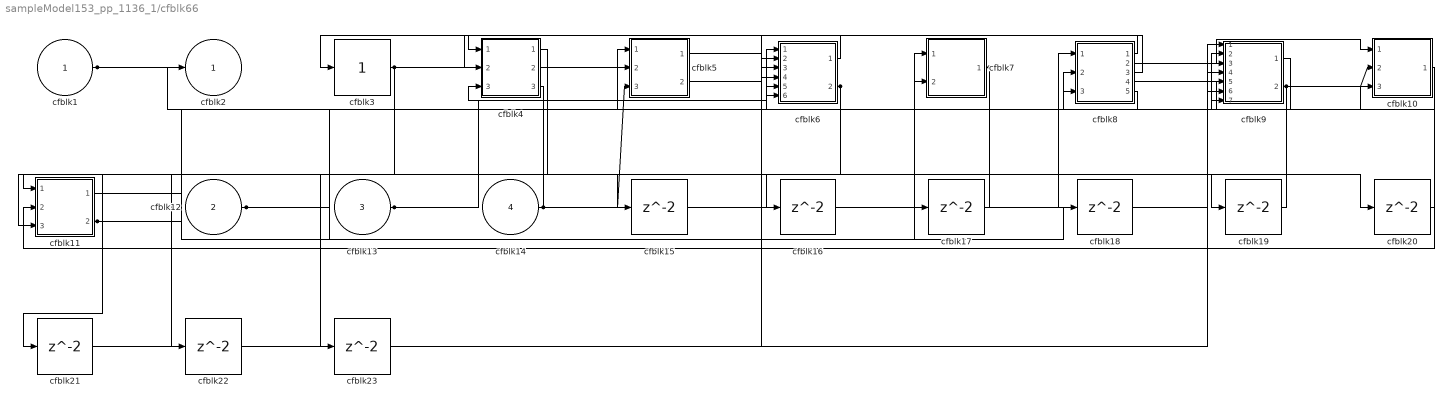
== system sampleModel153_pp_1136_1/cfblk66 ==
  cfblk1 : Inport
  cfblk12 : Inport  Port=2
  cfblk13 : Inport  Port=3
  cfblk14 : Inport  Port=4
  cfblk10 : Subsystem
  cfblk11 : Subsystem
  cfblk{15..23} (9 alike) : Delay  SampleTime=1
  cfblk3 : simulink/Math Operations/Slider Gain  gain=1  low=0  high=2
  cfblk4 : Subsystem
  cfblk5 : Subsystem
  cfblk6 : Subsystem
  cfblk7 : Subsystem
  cfblk8 : Subsystem
  cfblk9 : Subsystem
  cfblk2 : Outport
  wires:
  cfblk7/1(cfblk2) -> cfblk16/1, cfblk17/1
  cfblk13/1 -> cfblk6/1(cfblk1), cfblk9/2(cfblk11)
  cfblk8/1(cfblk2) -> cfblk3/1
  cfblk8/2(cfblk14) -> cfblk10/1(cfblk1)
  cfblk6/1(cfblk2) -> cfblk4/1(cfblk1)
  cfblk3/1 -> cfblk6/2(cfblk12), cfblk23/1
  cfblk9/1(cfblk2) -> cfblk8/2(cfblk12)
  cfblk1/1 -> cfblk2/1, cfblk9/5(cfblk14)
  cfblk9/2(cfblk17) -> cfblk10/2(cfblk10), cfblk6/5(cfblk15)
  cfblk12/1 -> cfblk7/1(cfblk1), cfblk9/7(cfblk16)
  cfblk8/3(cfblk15) -> cfblk4/2(cfblk13)
  cfblk6/2(cfblk17) -> cfblk11/1(cfblk1), cfblk22/1
  cfblk8/4(cfblk16) -> cfblk10/3(cfblk11)
  cfblk10/1(cfblk2) -> cfblk11/2(cfblk14)
  cfblk11/2(cfblk16) -> cfblk7/2(cfblk11), cfblk18/1
  cfblk4/1(cfblk2) -> cfblk11/3(cfblk15)
  cfblk4/2(cfblk15) -> cfblk5/1(cfblk1)
  cfblk8/5(cfblk17) -> cfblk5/2(cfblk14)
  cfblk14/1 -> cfblk5/3(cfblk15), cfblk4/3(cfblk14)
  cfblk11/1(cfblk2) -> cfblk15/1
  cfblk15/1 -> cfblk9/1(cfblk1)
  cfblk16/1 -> cfblk8/1(cfblk1)
  cfblk17/1 -> cfblk6/6(cfblk16)
  cfblk18/1 -> cfblk9/6(cfblk15)
  cfblk5/1(cfblk2) -> cfblk19/1
  cfblk19/1 -> cfblk8/3(cfblk13)
  cfblk5/2(cfblk16) -> cfblk20/1
  cfblk20/1 -> cfblk6/4(cfblk14)
  cfblk4/3(cfblk16) -> cfblk21/1
  cfblk21/1 -> cfblk6/3(cfblk13)
  cfblk22/1 -> cfblk9/3(cfblk12)
  cfblk23/1 -> cfblk9/4(cfblk13)

== system sampleModel153_pp_1136_1/cfblk67 ==
  cfblk1 : Inport
  cfblk6 : Inport  Port=2
  cfblk7 : Inport  Port=3
  cfblk3 : DiscreteIntegrator  ICPrevOutput=DiscIntNeverNeededParam  ICPrevScaledInput=DiscIntNeverNeededParam
  cfblk4 : Subsystem
  cfblk5 : Subsystem
  cfblk8 : Delay  SampleTime=1
  cfblk9 : Delay  SampleTime=1
  cfblk2 : Outport
  wires:
  cfblk6/1 -> cfblk5/1(cfblk1)
  cfblk1/1 -> cfblk4/1(cfblk1), cfblk4/5(cfblk10)
  cfblk3/1 -> cfblk5/2(cfblk8)
  cfblk4/1(cfblk2) -> cfblk3/1
  cfblk4/2(cfblk11) -> cfblk2/1
  cfblk7/1 -> cfblk4/2(cfblk7)
  cfblk5/1(cfblk2) -> cfblk8/1
  cfblk8/1 -> cfblk4/3(cfblk8)
  cfblk5/2(cfblk9) -> cfblk9/1
  cfblk9/1 -> cfblk4/4(cfblk9)

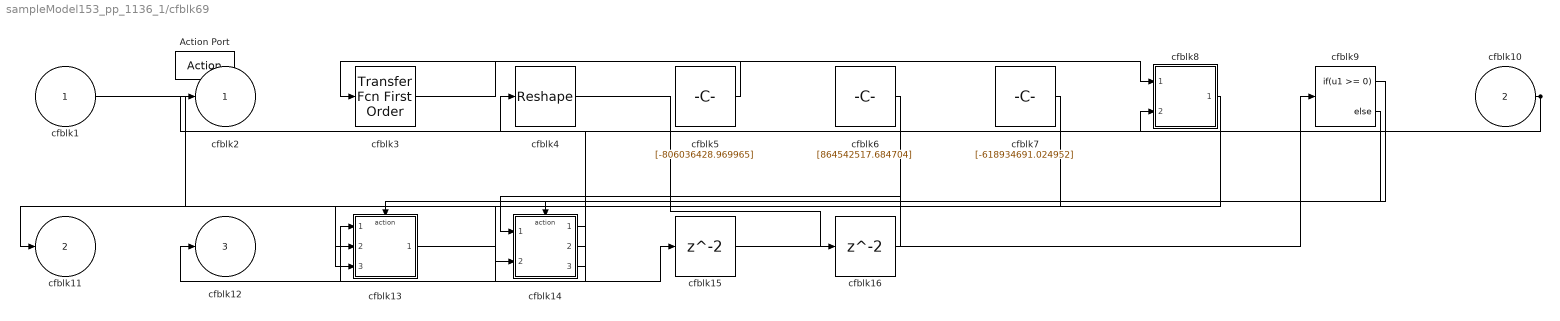
== system sampleModel153_pp_1136_1/cfblk69 ==
  cfblk1 : Inport
  cfblk10 : Inport  Port=2
  Action Port : ActionPort  ActionPortLabel=if(u1 >= 0)
  cfblk13 : Subsystem  TreatAsAtomicUnit=on
  cfblk14 : Subsystem  TreatAsAtomicUnit=on
  cfblk15 : Delay
  cfblk16 : Delay
  cfblk3 : simulink/Discrete/Transfer Fcn First Order  PoleZ=0.95  ICPrevOutput=0.0  DoSatur=off
  cfblk4 : Reshape
  cfblk5 : Constant  Value=[-806036428.969965]  SampleTime=1
  cfblk6 : Constant  Value=[864542517.684704]  SampleTime=1
  cfblk7 : Constant  Value=[-618934691.024952]  SampleTime=1
  cfblk8 : Subsystem
  cfblk9 : If  IfExpression=u1 >= 0  SampleTime=1
  cfblk2 : Outport
  cfblk11 : Outport  Port=2
  cfblk12 : Outport  Port=3
  wires:
  cfblk7/1 -> cfblk11/1
  cfblk5/1 -> cfblk3/1
  cfblk14/1(cfblk2) -> cfblk13/1(cfblk1)
  cfblk14/2(cfblk12) -> cfblk12/1
  cfblk14/3(cfblk13) -> cfblk4/1
  cfblk3/1 -> cfblk8/1(cfblk1)
  cfblk1/1 -> cfblk14/2(cfblk11)
  cfblk6/1 -> cfblk13/2(cfblk9)
  cfblk10/1 -> cfblk8/2(cfblk11), cfblk2/1
  cfblk8/1(cfblk2) -> cfblk13/3(cfblk10)
  cfblk9/1 -> cfblk13/Action
  cfblk9/2 -> cfblk14/Action
  cfblk13/1(cfblk2) -> cfblk15/1
  cfblk15/1 -> cfblk9/1
  cfblk4/1 -> cfblk16/1
  cfblk16/1 -> cfblk14/1(cfblk1)

== system sampleModel153_pp_1136_1/cfblk70 ==
  cfblk1 : Inport
  cfblk9 : Inport  Port=2
  Action Port : ActionPort  ActionPortLabel=else
  cfblk10 : Delay
  cfblk11 : Delay
  cfblk12 : Delay
  cfblk3 : Delay  ShowEnablePort=on
      settings: InputPortMap=u0,e6
  cfblk4 : Delay  DelayLengthSource=Input port
      settings: InputPortMap=u0,p1
  cfblk5 : Sum  Inputs=+
  cfblk6 : MinMax  Function=max  Inputs=3
  cfblk7 : Rounding
  cfblk8 : Subsystem
  cfblk2 : Outport
  wires:
  cfblk8/1(cfblk2) -> cfblk5/1, cfblk7/1
  cfblk6/1 -> cfblk4/1, cfblk8/2(cfblk5)
  cfblk9/1 -> cfblk4/2
  cfblk3/1 -> cfblk8/1(cfblk1), cfblk8/3(cfblk6), cfblk8/4(cfblk7)
  cfblk4/1 -> cfblk11/1, cfblk12/1
  cfblk1/1 -> cfblk3/2, cfblk6/3
  cfblk5/1 -> cfblk2/1
  cfblk7/1 -> cfblk10/1
  cfblk10/1 -> cfblk3/1
  cfblk11/1 -> cfblk6/1
  cfblk12/1 -> cfblk6/2

== system sampleModel153_pp_1136_1/cfblk76 ==
  emi_19 : Inport
  Action Port : ActionPort  ActionPortLabel=else
  cfblk76 : Delay  SampleTime=1
  emi_20 : Outport
  wires:
  emi_19/1 -> cfblk76/1
  cfblk76/1 -> emi_20/1

== system sampleModel153_pp_1136_1/cfblk77 ==
  emi_97 : Inport
  Action Port : ActionPort  ActionPortLabel=else
  cfblk77 : Delay  SampleTime=1
  emi_98 : Outport
  wires:
  emi_97/1 -> cfblk77/1
  cfblk77/1 -> emi_98/1

== system sampleModel153_pp_1136_1/emi_118 ==
  emi_125 : Inport
  Action Port : ActionPort  ActionPortLabel=if(-1.115962e+09 > u1)
  emi_122 : Trigonometry
  emi_123 : Abs
  emi_124 : Math  SaturateOnIntegerOverflow=on
  emi_126 : Outport
  wires:
  emi_125/1 -> emi_122/1
  emi_122/1 -> emi_123/1
  emi_123/1 -> emi_124/1

== system sampleModel153_pp_1136_1/emi_21 ==
  emi_28 : Inport
  Action Port : ActionPort  ActionPortLabel=if(-1.237869e+09 > u1)
  emi_25 : MinMax  SampleTime=1
  emi_26 : MinMax  SampleTime=1
  emi_27 : MinMax  SampleTime=1
  emi_29 : Outport
  wires:
  emi_28/1 -> emi_25/1
  emi_25/1 -> emi_26/1
  emi_26/1 -> emi_27/1

== system sampleModel153_pp_1136_1/emi_3 ==
  emi_10 : Inport
  Action Port : ActionPort  ActionPortLabel=if(-9.023192e+10 > u1)
  emi_7 : MinMax  SampleTime=1
  emi_8 : Math  SampleTime=1  SaturateOnIntegerOverflow=on
  emi_9 : Trigonometry  SampleTime=1
  emi_11 : Outport
  wires:
  emi_10/1 -> emi_7/1
  emi_7/1 -> emi_8/1
  emi_8/1 -> emi_9/1

== system sampleModel153_pp_1136_1/emi_42 ==
  emi_49 : Inport
  Action Port : ActionPort  ActionPortLabel=if(0 > u1)
  emi_46 : Abs  SampleTime=1
  emi_47 : MinMax  SampleTime=1
  emi_48 : Trigonometry  SampleTime=1
  emi_50 : Outport
  wires:
  emi_49/1 -> emi_46/1
  emi_46/1 -> emi_47/1
  emi_47/1 -> emi_48/1

== system sampleModel153_pp_1136_1/emi_60 ==
  emi_67 : Inport
  Action Port : ActionPort  ActionPortLabel=if(0 > u1)
  emi_64 : Math  SaturateOnIntegerOverflow=on
  emi_65 : Trigonometry
  emi_66 : Gain
  emi_68 : Outport
  wires:
  emi_67/1 -> emi_64/1
  emi_64/1 -> emi_65/1
  emi_65/1 -> emi_66/1

== system sampleModel153_pp_1136_1/emi_81 ==
  emi_88 : Inport
  Action Port : ActionPort  ActionPortLabel=if(-Inf > u1)
  emi_85 : Trigonometry
  emi_86 : MinMax
  emi_87 : Trigonometry
  emi_89 : Outport
  wires:
  emi_88/1 -> emi_85/1
  emi_85/1 -> emi_86/1
  emi_86/1 -> emi_87/1

== system sampleModel153_pp_1136_1/emi_99 ==
  emi_106 : Inport
  Action Port : ActionPort  ActionPortLabel=if(0 > u1)
  emi_103 : MinMax  SampleTime=1
  emi_104 : Trigonometry  SampleTime=1
  emi_105 : MinMax  SampleTime=1
  emi_107 : Outport
  wires:
  emi_106/1 -> emi_103/1
  emi_103/1 -> emi_104/1
  emi_104/1 -> emi_105/1
